simulink model "Nao_linear"  (R2020b)
settings: Solver=VariableStepAuto  StartTime=0.0  StopTime=300  FixedStep=10^-3  RelTol=1e-3
values from neighbouring files (symbols this model uses):
  Heq = 5    [Moodle.m]    (also in Resposta_ao_escalao_Gclr_Ex_3_5.m; Resposta_ao_escalao_Gclr_Ex_4_7.m)
settings Model: Creator=rodsc  LastModifiedBy=rodsc

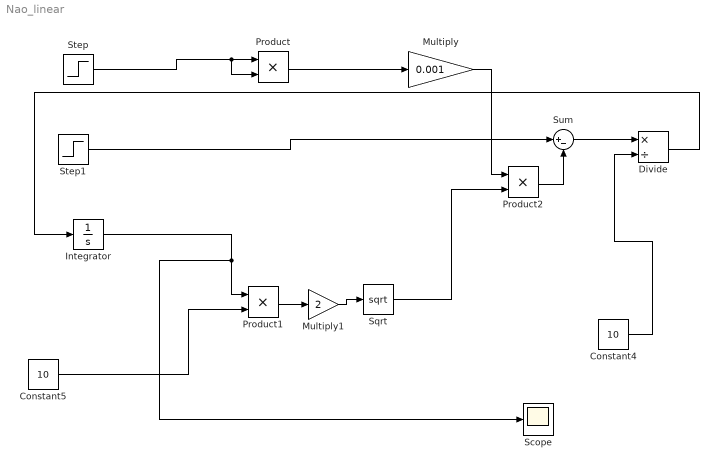
== system Nao_linear ==
  Constant4 : Constant  Value=10
  Constant5 : Constant  Value=10
  Divide : Product  Inputs=*/
  Integrator : Integrator  InitialCondition=Heq
  Multiply : Gain  Gain=0.001
  Multiply1 : Gain  Gain=2
  Product : Product
  Product1 : Product
  Product2 : Product
  Scope : Scope
  Sqrt : Sqrt  SaturateOnIntegerOverflow=on
  Step : Step  After=20  SampleTime=0
  Step1 : Step  SampleTime=0
  Sum : Sum  Inputs=|+-
  wires:
  Product/1 -> Multiply/1
  Constant5/1 -> Product1/2
  Product1/1 -> Multiply1/1
  Multiply1/1 -> Sqrt/1
  Sqrt/1 -> Product2/2
  Multiply/1 -> Product2/1
  Product2/1 -> Sum/2
  Sum/1 -> Divide/1
  Constant4/1 -> Divide/2
  Divide/1 -> Integrator/1
  Integrator/1 -> Product1/1, Scope/1
  Step/1 -> Product/2, Product/1
  Step1/1 -> Sum/1
